simulink model "Controller_PIL"  (R2023b)
settings: Solver=FixedStepDiscrete  StartTime=0.0  StopTime=0.5  RelTol=1e-3  EnableMultiTasking=on
libraries: pil_lib x1
settings Model: Creator=Tefilus  LastModifiedBy=Tefilus
settings SolverCC: AlgebraicLoopSolver=TrustRegion
settings OptimizationCC: DefaultParameterBehavior=Inlined  DefaultUnderspecifiedDataType=single  EnhancedBackFolding=on  PassReuseOutputArgsAs=Individual arguments  MaxStackSize=1024  OptimizeBlockOrder=speed  DifferentSizesBufferReuse=on  OptimizationCustomize=off  DenormalBehavior=FlushToZero  EfficientTunableParamExpr=on
settings DebuggingCC: ParameterPrecisionLossMsg=none  ParameterTunabilityLossMsg=error  UnconnectedInputMsg=warning  UnconnectedOutputMsg=warning  UnconnectedLineMsg=warning
settings HardwareCC: ProdBitPerChar=16  ProdBitPerInt=16  ProdBitPerPointer=32  ProdBitPerSizeT=32  ProdBitPerPtrDiffT=32  ProdLargestAtomicInteger=Integer  ProdLargestAtomicFloat=None  ProdWordSize=16  ProdLongLongMode=on  ProdHWDeviceType=Texas Instruments->C2000  HardwareBoardFeatureSet=SoCBlockset
settings ModelReferenceCC: EnableRefExpFcnMdlSchedulingChecks=on  ModelReferenceNumInstancesAllowed=Single
settings SFSimCC: MATLABDynamicMemAlloc=off
settings RTWCC: Description=Embedded Coder  SystemTargetFile=ert.tlc  HardwareBoard=TI Piccolo F28069M LaunchPad  TemplateMakefile=ert_default_tmf  Toolchain=Texas Instruments Code Composer Studio (C2000)  CreateSILPILBlock=PIL  CodeExecutionProfiling=on  CodeProfilingInstrumentation=coarse  DLArmComputeVersion=19.05
settings CodeAppCC: ForceParamTrailComments=on  IgnoreCustomStorageClasses=off  OperatorAnnotations=on  SimulinkDataObjDesc=on  SFDataObjDesc=on  InsertBlockDesc=on
settings ERTTargetCC: CodeReplacementLibrary=TI C28x  ExtModeTransport=4  ExtModeStaticAlloc=on  ExtModeAutomaticAllocSize=off  ExtModeStaticAllocSize=2000  ExtModeMexFile=ext_xcp  ExtModeIntrfLevel=Level2 - Open

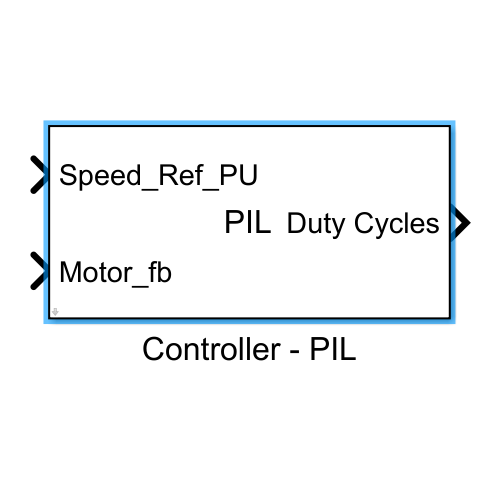
[thumbnail: Simulink's stored preview of the top-level diagram]
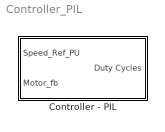
== system Controller_PIL ==
  Controller - PIL : Subsystem  DialogController=pil_create_dialog  LoadFcn=|
      | try
      |    if ~strcmp(rtw.pil.getPILVersion, '23.2 (R2023b)_15')
      |       set_param(gcb, 'DialogController', '');
      |       set_param(gcb, 'DialogControllerArgs', '');
      |    end
      | catch e
      |       set_param(gcb, 'DialogController', '');
      |       set_param(gcb, 'DialogControllerArgs', '');
      | end
      mask help: PIL:pil:XILBlockMaskDesc
      mask Display: disp('PIL');

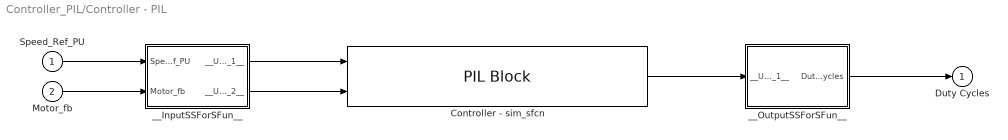
== system Controller_PIL/Controller - PIL ==
  Speed_Ref_PU : Inport
  Motor_fb : Inport  Port=2
  Controller - sim_sfcn : pil_lib/PIL Block  SimulationMode=PIL  IsTopModelPIL=off  CodeDir=Controller_ert_rtw  AnchorDir=E:\GiaotrinhDH\DATN\exampleSIL_PIL_MIL_HIL\FOC_QEP  ConfigName=Texas Instruments C2000 Base  XrelIsTopModelCode=on  XrelIsReusable=off  XrelDWorkNames={}  XrelDWorkTypes={}  XrelModelArgVals={}  XrelOrderedParamNames={}
  __InputSSForSFun__ : Subsystem
  __OutputSSForSFun__ : Subsystem
  Duty Cycles : Outport
  wires:
  Speed_Ref_PU/1 -> __InputSSForSFun__/1(Speed_Ref_PU)
  Motor_fb/1 -> __InputSSForSFun__/2(Motor_fb)
  __InputSSForSFun__/1(__UniqueOutportName__1__) -> Controller - sim_sfcn/1
  __InputSSForSFun__/2(__UniqueOutportName__2__) -> Controller - sim_sfcn/2
  Controller - sim_sfcn/1 -> __OutputSSForSFun__/1(__UniqueInportName__1__)
  __OutputSSForSFun__/1(Duty Cycles) -> Duty Cycles/1

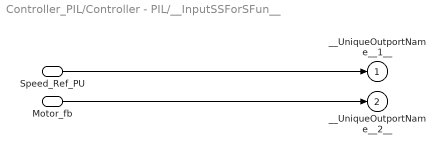
== system Controller_PIL/Controller - PIL/__InputSSForSFun__ ==
  Speed_Ref_PU : Inport
  Motor_fb : Inport  Port=2
  __UniqueOutportName__1__ : Outport
  __UniqueOutportName__2__ : Outport  Port=2
  wires:
  Speed_Ref_PU/1 -> __UniqueOutportName__1__/1
  Motor_fb/1 -> __UniqueOutportName__2__/1

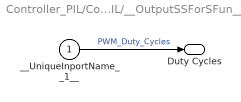
== system Controller_PIL/Controller - PIL/__OutputSSForSFun__ ==
  __UniqueInportName__1__ : Inport
  Duty Cycles : Outport
  wires:
  __UniqueInportName__1__/1 -> Duty Cycles/1  "PWM_Duty_Cycles"
